simulink model "Pedirtiempo"  (R2020b)
settings: Solver=VariableStepAuto  StartTime=0.0  StopTime=10.0  RelTol=1e-3
settings Model: Creator=cacha  LastModifiedBy=cacha

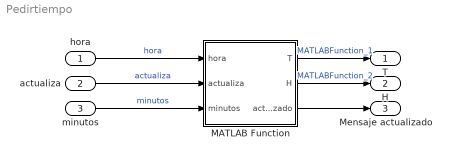
== system Pedirtiempo ==
  "hora " : Inport  OutMin=0  OutMax=72  OutDataTypeStr=double  PortDimensions=1
  "actualiza " : Inport  Port=2  OutMin=0  OutMax=1  OutDataTypeStr=double  PortDimensions=1
  minutos : Inport  Port=3  OutMin=0  OutMax=30  OutDataTypeStr=double  PortDimensions=1
  MATLAB Function : MATLAB Function  TreatAsAtomicUnit=on
  T : Outport  SignalName=T  OutMin=0  OutMax=35  OutDataTypeStr=double  PortDimensions=1
      settings: MustResolveToSignalObject=on
  H : Outport  Port=2  SignalName=H  OutMin=0  OutMax=1  OutDataTypeStr=double  PortDimensions=1
      settings: MustResolveToSignalObject=on
  Mensaje actualizado : Outport  Port=3  SignalName=H  OutMin=0  OutMax=1  OutDataTypeStr=double  PortDimensions=1
      settings: MustResolveToSignalObject=on
  wires:
  MATLAB Function/1(T) -> T/1  "MATLABFunction_1"
  MATLAB Function/2(H) -> H/1  "MATLABFunction_2"
  "hora "/1 -> MATLAB Function/1(hora)  "hora"
  "actualiza "/1 -> MATLAB Function/2(actualiza)  "actualiza"
  minutos/1 -> MATLAB Function/3(minutos)  "minutos"
  MATLAB Function/3(actualizado) -> Mensaje actualizado/1

== matlab function Pedirtiempo/MATLAB Function ==
  data: hora input; T output; actualiza input; H output; minutos input; actualizado output
function [T,H,actualizado] = fcn(hora,actualiza,minutos)

persistent x0 

if hora==24 || actualiza == 1 
%significará que ha pasado de día o cada 
%media hora, o se ha pedido actualizar por el usuario

if isempty(x0)
   x0=1651255;
end
m=2^31;
x0=rem(314159269*x0+453806245,m);
uniforme=x0/m;

    T = uniforme * 35;
    disp('La temperatura de hoy es de');
%     disp(T);

    H = uniforme;
    disp('La humedad de hoy es de');
%     disp(H);
    
    T1 = uniforme * 35;
    disp('La temperatura de mañana es de');
    disp(T1);

    H1 = uniforme;
    disp('La humedad de mañana es de');
    disp(H1);
    
    T2 = uniforme * 35;
    disp('La temperatura de pasado mañana es de');
    disp(T2);

    H2 = uniforme;
    disp('La humedad de pasado mañana es de');
    disp(H2);  
    hora = 0;
    actualizado = 1;
else 
    T = 0;
    H = 0;
    actualizado = 0;
end
if minutos == 30
  if isempty(x0)
  x0=1651255;
  end
m=2^31;
x0=rem(314159269*x0+453806245,m);
uniforme=x0/m;

    T = uniforme * 35;
    H = uniforme;
    actualizado = 1;
else
    actualizao = 0;
end
end
